simulink model "task5_lab2"  (R2020b)
settings: Solver=VariableStepAuto  StartTime=1  StopTime=40  RelTol=1e-3  EnableMultiTasking=on
settings Model: Creator=JackShen  LastModifiedBy=mluser
settings DataIOCC: LimitDataPoints=on  ReturnWorkspaceOutputs=off
settings OptimizationCC: LifeSpan=inf
settings DebuggingCC: AllowSymbolicDim=off  SFUnexpectedBacktrackingDiag=warning  SFNoUnconditionalDefaultTransitionDiag=warning  SFExecutionAtInitializationDiag=none  ArithmeticOperatorsInVariantConditions=warning
settings ModelReferenceCC: PropagateSignalLabelsOutOfModel=off
settings SFSimCC: SimUseLocalCustomCode=off  CustomCodeUndefinedFunction=UseInterfaceOnly
settings RTWCC: RTWUseLocalCustomCode=off
settings CodeAppCC: StateflowObjectComments=on
settings GRTTargetCC: TargetLangStandard=C89/C90 (ANSI)
settings ConfigComp: CovMetricSettings=dw  CovSaveCumulativeToWorkspaceVar=on  CovSaveSingleToWorkspaceVar=on  CovExternalEMLEnable=off

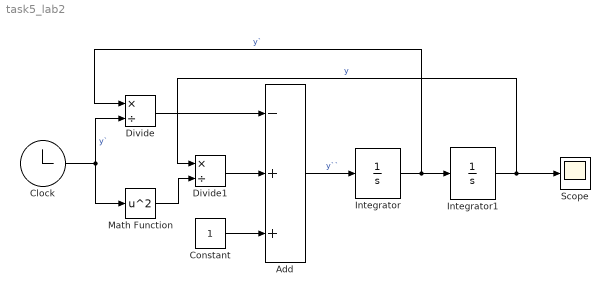
== system task5_lab2 ==
  Add : Sum  Inputs=-++
  Clock : Clock
  Constant : Constant
  Divide : Product  Inputs=*/
  Divide1 : Product  Inputs=*/
  Integrator : Integrator  InitialCondition=3
  Integrator1 : Integrator  InitialCondition=6
  Math Function : Math  Operator=square  SignedPower=on  SaturateOnIntegerOverflow=on
  Scope : Scope
  wires:
  Add/1 -> Integrator/1  "y``"
  Divide/1 -> Add/1
  Divide1/1 -> Add/2
  Constant/1 -> Add/3
  Math Function/1 -> Divide1/2
  Clock/1 -> Divide/2, Math Function/1  "y`"
  Integrator/1 -> Divide/1, Integrator1/1  "y`"
  Integrator1/1 -> Divide1/1, Scope/1  "y"
